simulink model "pwm_thesis"  (R2018a)
settings: Solver=VariableStepAuto  StartTime=0.0  StopTime=5  MaxStep=0.01  RelTol=1e-3
libraries: powerlib x75, simulink x17, powerlib_meascontrol x1
settings Model: Creator=buzaevfedor  LastModifiedBy=buzaevfedor
settings SolverCC: ZeroCrossAlgorithm=Adaptive
settings DebuggingCC: MaxConsecutiveZCsMsg=none  MaskedZcDiagnostic=none

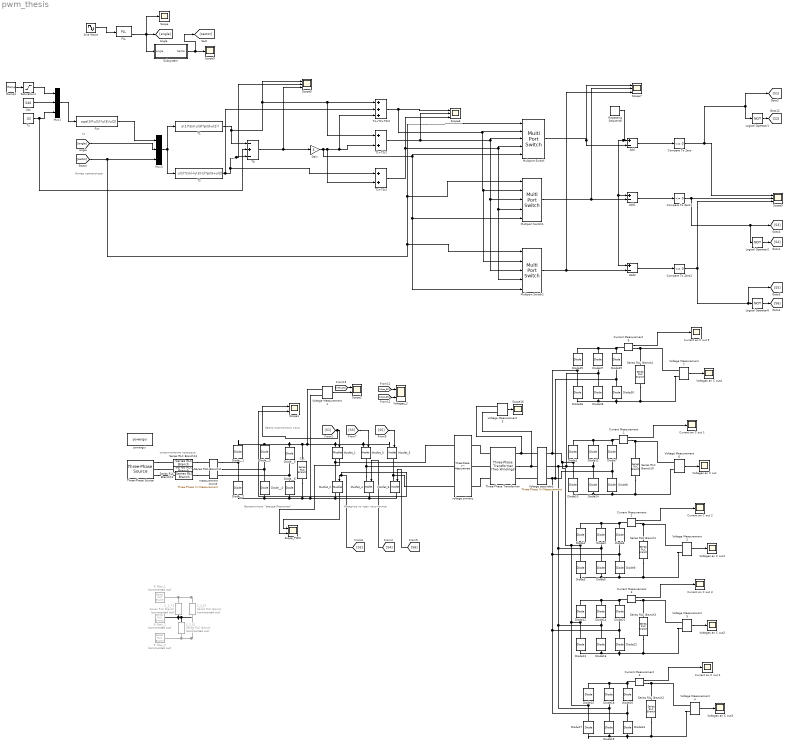
== system pwm_thesis ==
  note: Номер транзистора
  note: wt
  note: Выпрямитель "звезда-Ларионов"
  note: Звено постоянного тока
  note: Инвертор из трех полумостов
  note: сопротивление проводов
  Add : Sum  Inputs=+-
  Add1 : Sum  Inputs=+-
  Add2 : Sum  Inputs=+-
  C_1 : powerlib/Elements/Series RLC Branch  LConnTagsString=__new0  RConnTagsString=__new0  BranchType=C  Resistance=1  Inductance=1e-3  SetiL0=off  InitialCurrent=0  Capacitance=1000e-6  Setx0=off  InitialVoltage=0  Measurements=Branch voltage and current
  C_1_f 2 : powerlib/Elements/Series RLC Branch  Commented=on  LConnTagsString=__new0  RConnTagsString=__new0  BranchType=C  Resistance=1  Inductance=1e-3  SetiL0=off  InitialCurrent=0  Capacitance=1100e-8  Setx0=off  InitialVoltage=0  Measurements=None
  C_2_f2 : powerlib/Elements/Series RLC Branch  Commented=on  LConnTagsString=__new0  RConnTagsString=__new0  BranchType=C  Resistance=1  Inductance=1e-3  SetiL0=off  InitialCurrent=0  Capacitance=1100e-8  Setx0=off  InitialVoltage=0  Measurements=None
  C_3_f2 : powerlib/Elements/Series RLC Branch  Commented=on  LConnTagsString=__new0  RConnTagsString=__new0  BranchType=C  Resistance=1  Inductance=1e-3  SetiL0=off  InitialCurrent=0  Capacitance=1100e-8  Setx0=off  InitialVoltage=0  Measurements=None
  Compare To Zero : simulink/Logic and Bit Operations/Compare To Zero  relop=<=  OutDataTypeStr=boolean
  Compare To Zero1 : simulink/Logic and Bit Operations/Compare To Zero  relop=<=  OutDataTypeStr=boolean
  Compare To Zero2 : simulink/Logic and Bit Operations/Compare To Zero  relop=<=  OutDataTypeStr=boolean
  Current Measurement{1..5} (5 alike) : powerlib/Measurements/Current Measurement  PhasorSimulation=off  OutputType=Complex  PSBequivalent=0
  Current an C out {1..5} (5 alike) : Scope
  Diode{1..30} (30 alike) : powerlib/Power Electronics/Diode  Ron=0.001  Lon=0  Vf=0.8  IC=0  UseSnubber=0  Rs=500  Cs=250e-9  Measurements=off
  Diode__{1..6} (6 alike) : powerlib/Power Electronics/Diode  Ron=0.001  Lon=0  Vf=0.8  IC=0  UseSnubber=0  Rs=500  Cs=250e-9  Measurements=off
  Fcn : Fcn  Expr=sqrt(3)*u(1)*u(3)/u(2)
  Gain : Gain  Gain=.5
  Logical Operator1 : Logic  Operator=NOT  AllPortsSameDT=off  OutDataTypeStr=boolean
  Logical Operator2 : Logic  Operator=NOT  AllPortsSameDT=off  OutDataTypeStr=boolean
  Logical Operator6 : Logic  Operator=NOT  AllPortsSameDT=off  OutDataTypeStr=boolean
  Mosfet_1 : powerlib/Power Electronics/Mosfet  Ron=0.1  Lon=0  Rd=0.01  Vfd=0  IC=0  Rs=1e5  Cs=inf  Measurements=on
  Mosfet_2 : powerlib/Power Electronics/Mosfet  Ron=0.1  Lon=0  Rd=0.01  Vfd=0  IC=0  Rs=1e5  Cs=inf  Measurements=on
  Mosfet_{3..6} (4 alike) : powerlib/Power Electronics/Mosfet  Ron=0.1  Lon=0  Rd=0.01  Vfd=0  IC=0  Rs=1e5  Cs=inf  Measurements=off
  Multiport Switch : MultiPortSwitch  DataPortOrder=Specify indices  Inputs=4  DataPortIndices={[1,6],2,5,[3,4]}  DiagnosticForDefault=Warning
  Multiport Switch1 : MultiPortSwitch  DataPortOrder=Specify indices  Inputs=4  DataPortIndices={[2,3],4,1,[5,6]}  DiagnosticForDefault=Warning
  Multiport Switch2 : MultiPortSwitch  DataPortOrder=Specify indices  Inputs=4  DataPortIndices={[4,5],6,3,[1,2]}  DiagnosticForDefault=Warning
  Mux1 : Mux  Inputs=3
  Mux3 : Mux  Inputs=3
  PLL : powerlib_meascontrol/PLL/PLL  Fmin=45  Par_Init=[0, 50]  ParK=[180, 3200, 1]  TcD=1e-4  MaxRateChangeFreq=12  FilterCutOffFreq=25  Ts=0  AGC=on
      settings: SourceProductName=Simscape Power Systems  SourceProductBaseCode=PS
  R filter_1 : powerlib/Elements/Series RLC Branch  Commented=on  LConnTagsString=__new0  RConnTagsString=__new0  BranchType=R  Resistance=80  Inductance=1e-3  SetiL0=off  InitialCurrent=0  Capacitance=1e-6  Setx0=off  InitialVoltage=0  Measurements=None
  R filter_2 : powerlib/Elements/Series RLC Branch  Commented=on  LConnTagsString=__new0  RConnTagsString=__new0  BranchType=R  Resistance=80  Inductance=1e-3  SetiL0=off  InitialCurrent=0  Capacitance=1e-6  Setx0=off  InitialVoltage=0  Measurements=None
  R filter_3 : powerlib/Elements/Series RLC Branch  Commented=on  LConnTagsString=__new0  RConnTagsString=__new0  BranchType=R  Resistance=80  Inductance=1e-3  SetiL0=off  InitialCurrent=0  Capacitance=1e-6  Setx0=off  InitialVoltage=0  Measurements=None
  Ramp1 : simulink/Sources/Ramp  slope=55  start=0  InitialOutput=0
  Repeating Sequence : simulink/Sources/Repeating Sequence  rep_seq_t=[0 .001]  rep_seq_y=[0 .02]
  Saturation1 : Saturate  UpperLimit=220
  Scope : Scope
  Scope1 : Scope  NumInputPorts=2
  Scope16 : Scope
  Scope2 : Scope  NumInputPorts=2
  Scope3 : Scope
  Scope{5..7,9} (4 alike) : Scope  NumInputPorts=3
  Scope_PWM : Scope  NumInputPorts=2
  Series RLC Branch{1..4,10} (5 alike) : powerlib/Elements/Series RLC Branch  LConnTagsString=__new0  RConnTagsString=__new0  BranchType=C  Resistance=1  Inductance=1e-3  SetiL0=off  InitialCurrent=0  Capacitance=12e-3  Setx0=off  InitialVoltage=0  Measurements=Branch voltage and current
  Series RLC Branch11 : powerlib/Elements/Series RLC Branch  LConnTagsString=__new0  RConnTagsString=__new0  BranchType=RL  Resistance=1  Inductance=1e-3  SetiL0=off  InitialCurrent=0  Capacitance=1e-6  Setx0=off  InitialVoltage=0  Measurements=None
  Series RLC Branch12 : powerlib/Elements/Series RLC Branch  LConnTagsString=__new0  RConnTagsString=__new0  BranchType=RL  Resistance=1  Inductance=1e-3  SetiL0=off  InitialCurrent=0  Capacitance=1e-6  Setx0=off  InitialVoltage=0  Measurements=None
  Series RLC Branch13 : powerlib/Elements/Series RLC Branch  LConnTagsString=__new0  RConnTagsString=__new0  BranchType=RL  Resistance=1  Inductance=1e-3  SetiL0=off  InitialCurrent=0  Capacitance=1e-6  Setx0=off  InitialVoltage=0  Measurements=None
  Sine Wave : Sin  Frequency=2*pi*50  SampleTime=0
  Subsystem : Subsystem
  T0 : Sum  Inputs=-+-
  T1 : Fcn  Expr=u(1)*sin(u(3)*pi/3-u(2))
  T1+T0/2 : Sum  Inputs=2
  T1+T2+T0/2 : Sum  Inputs=+++
  T2 : Fcn  Expr=u(1)*sin(-(u(3)-1)*pi/3+u(2))
  T2+T0/2 : Sum  Inputs=2
  Three-Phase Transformer : powerlib/Elements/Three-Phase Transformer (Two Windings)  Winding1Connection=Yg  Winding2Connection=Yg  CoreType=Three single-phase transformers  SetSaturation=off  Hysteresis=off  DataFile='hysteresis'  SetInitialFlux=off  Measurements=None  UNITS=SI  NominalPower=[8549523 , 50 ]  Winding1=[7.35e+05 0.069 1.108e-03]  Winding2=[14.15e+05 8.86e-4 0.09e-03]  Rm=5980.4  Lm=19.93  L0=0.5  Saturation=[0 0;0.66653 1910.3;277.72 2419.7]  InitialFluxes=[1273.5 -1273.5 1114.3]  MoreParameters=off  BreakLoop=off  DataType=on  TransfoNumber=1
  Three-Phase Source : powerlib/Electrical Sources/Three-Phase Source  InternalConnection=Yg  VoltagePhases=on  Voltage=380  PhaseAngle=0  Voltage_phases=[380 380 380]/sqrt(3)  PhaseAngles_phases=[0 -120 +120]  Frequency=50  NonIdealSource=off  SpecifyImpedance=off  Resistance=0.8929  Inductance=16.58e-3  ShortCircuitLevel=100e6  BaseVoltage=25e3  XRratio=7  BusType=swing  Pref=10e3  Qref=0  Prefabc=[10e3, 10e3, 10e3]  Qrefabc=[0, 0, 0]  Qmin=-inf  Qmax=inf
  Tz : Constant  Value=.02
  Udc : Constant  Value=540
  Voltage Measurement{1..7} (7 alike) : powerlib/Measurements/Voltage Measurement  PhasorSimulation=off  OutputType=Complex  PSBequivalent=0
  Voltage secondary : powerlib/Measurements/Three-Phase V-I Measurement  VoltageMeasurement=phase-to-phase  SetLabelV=on  LabelV=Vabc_B3  Vpu=off  VpuLL=off  CurrentMeasurement=yes  SetLabelI=on  LabelI=Iabc_B3  Ipu=off  Pbase=225e3  Vbase=2400  OutputType=Complex  PhasorSimulation=off  PSBequivalent=0
  Voltages an C out{,1..4} (5 alike) : Scope
  Voltages_2 : Scope  NumInputPorts=2
  measurement source : powerlib/Measurements/Three-Phase V-I Measurement  VoltageMeasurement=phase-to-phase  SetLabelV=on  LabelV=Vabc_B1  Vpu=off  VpuLL=off  CurrentMeasurement=yes  SetLabelI=on  LabelI=Iabc_B1  Ipu=off  Pbase=225e3  Vbase=2400  OutputType=Complex  PhasorSimulation=off  PSBequivalent=0
  powergui : powerlib/powergui  Priority=1  SimulationMode=Continuous  SampleTime=50e-6  frequency=60  Iterations=50  frequencyindice=50  Pbase=100e6  ErrMax=1e-4  UnitsV=kV  UnitsW=MW  buscounter=0  FunctionMessages=off  echomessages=off  EnableUseOfTLC=off  CurrentSourceSwitches=off  DisableSnubberDevices=off  DisableRonSwitches=off  DisableVfSwitches=off  DisplayEquations=off  SolverType=Tustin/Backward Euler (TBE)  Interpol=off  ExternalGateDelay=off  methode=off  Ts=100  x0status=blocks  SPID=on  SwTol=0  HookPort=off  RestoreLinks=warning  ResistiveCurrentMeasurement=off  Frange=[0:2:500]  Ylog=off  Xlog=on  ShowGrid=off  save=off  variable=ZData  structure=0  ZoomFFT=off  StartTime=0.0  cycles=1  DisplayStyle=1  fundamental=60  FreqAxis=off  MaxFrequency=1000  frequencyindicesteady=1  RmsSteady=1  display=off
  "voltage primary " : powerlib/Measurements/Three-Phase V-I Measurement  VoltageMeasurement=phase-to-phase  SetLabelV=on  LabelV=Vabc_B2  Vpu=off  VpuLL=off  CurrentMeasurement=yes  SetLabelI=on  LabelI=Iabc_B2  Ipu=off  Pbase=225e3  Vbase=2400  OutputType=Complex  PhasorSimulation=off  PSBequivalent=0
  wires:
  Voltage Measurement3/1 -> Scope16/1
  Voltage Measurement6/1 -> Voltages an C out/1
  [Vabc_B3] -> Voltages_2/2
  [Vabc_B2] -> Voltages_2/1
  [S6] -> Mosfet_6/1
  [S2] -> Scope1/2, Mosfet_2/1
  [S3] -> Mosfet_3/1
  [S5] -> Mosfet_5/1
  [S1] -> Scope1/1, Mosfet_1/1
  Voltage Measurement1/1 -> Scope2/2
  [Vabc_B1] -> Scope2/1
  Mosfet_1/1 -> Scope_PWM/2
  Mosfet_2/1 -> Scope_PWM/1
  Current Measurement1/1 -> Current an C out 1/1
  Tz/1 -> T0/2, Mux1/3
  Compare To Zero1/1 -> Logical Operator2/1, [S3], Scope9/2
  Add/1 -> Compare To Zero/1
  Udc/1 -> Mux1/2
  Sine Wave/1 -> PLL/1
  Repeating Sequence/1 -> Add2/1, Add1/1, Add/1
  Multiport Switch2/1 -> Add2/2, Scope7/3
  Mux3/1 -> T2/1, T1/1
  T1+T0/2/1 -> Multiport Switch2/3, Multiport Switch1/3, Multiport Switch/3, Scope6/2
  Compare To Zero2/1 -> Scope9/3, [S5], Logical Operator6/1
  Gain/1 -> Multiport Switch2/5, Multiport Switch1/5, Multiport Switch/5, T2+T0/2/2, T1+T0/2/2, T1+T2+T0/2/3
  Multiport Switch/1 -> Add/2, Scope7/1
  Logical Operator1/1 -> [S2]
  T1/1 -> T1+T2+T0/2/1, T1+T0/2/1, Scope5/1, T0/1
  Fcn/1 -> Mux3/1
  Logical Operator6/1 -> [S6]
  Multiport Switch1/1 -> Add1/2, Scope7/2
  PLL/2 -> Scope/1, Subsystem/1(angle), [angle]
  [sector] -> Multiport Switch2/1, Multiport Switch1/1, Multiport Switch/1, Mux3/3
  T2/1 -> T1+T2+T0/2/2, T2+T0/2/1, Scope5/2, T0/3
  Subsystem/1(Sector) -> [sector], Scope3/1
  Add1/1 -> Compare To Zero1/1
  Logical Operator2/1 -> [S4]
  Mux1/1 -> Fcn/1
  Compare To Zero/1 -> Logical Operator1/1, [S1], Scope9/1
  [angle] -> Mux3/2
  T2+T0/2/1 -> Multiport Switch2/4, Multiport Switch1/4, Multiport Switch/4, Scope6/3
  T1+T2+T0/2/1 -> Multiport Switch2/2, Multiport Switch1/2, Multiport Switch/2, Scope6/1
  Add2/1 -> Compare To Zero2/1
  T0/1 -> Scope5/3, Gain/1
  [S4] -> Mosfet_4/1
  Ramp1/1 -> Saturation1/1
  Saturation1/1 -> Mux1/1
  Current Measurement2/1 -> Current an C out 2/1
  Voltage Measurement2/1 -> Voltages an C out1/1
  Voltage Measurement4/1 -> Voltages an C out3/1
  Current Measurement4/1 -> Current an C out 4/1
  Current Measurement3/1 -> Current an C out 3/1
  Voltage Measurement5/1 -> Voltages an C out2/1
  Current Measurement5/1 -> Current an C out 5/1
  Voltage Measurement7/1 -> Voltages an C out4/1
  connections:
  Diode8/LConn1 -- Diode10/LConn1 -- Diode24/LConn1 -- Voltage Measurement6/LConn2 -- Series RLC Branch10/RConn1
  Diode15/LConn1 -- Diode25/LConn1 -- Diode26/RConn1 -- Voltage secondary/RConn1 -- Diode10/RConn1 -- Diode1/LConn1 -- Diode2/LConn1 -- Diode3/RConn1 -- Diode12/LConn1 -- Diode13/RConn1 -- Diode17/RConn1
  Diode__6/RConn1 -- measurement source/RConn3 -- Diode__5/LConn1
  Mosfet_6/RConn1 -- Diode__2/LConn1 -- Diode__4/LConn1 -- Diode__6/LConn1 -- C_1/RConn1 -- Voltage Measurement1/LConn2 -- Mosfet_2/RConn1 -- Mosfet_4/RConn1
  Diode1/RConn1 -- Current Measurement1/LConn1 -- Diode7/RConn1 -- Diode11/RConn1
  Diode18/LConn1 -- Voltage secondary/RConn2 -- Diode27/LConn1 -- Diode28/RConn1 -- Diode24/RConn1 -- Diode11/LConn1 -- Diode4/LConn1 -- Diode5/RConn1 -- Diode14/LConn1 -- Diode16/RConn1 -- Diode19/RConn1
  Diode__5/RConn1 -- C_1/LConn1 -- Mosfet_1/LConn1 -- Mosfet_3/LConn1 -- Mosfet_5/LConn1 -- Voltage Measurement1/LConn1 -- Diode__1/RConn1 -- Diode__3/RConn1
  Voltage Measurement3/LConn2 -- Three-Phase Transformer/RConn2 -- Voltage secondary/LConn2
  Diode__4/RConn1 -- measurement source/RConn2 -- Diode__3/LConn1
  Voltage Measurement3/LConn1 -- Three-Phase Transformer/RConn1 -- Voltage secondary/LConn1
  Diode__1/LConn1 -- measurement source/RConn1 -- Diode__2/RConn1
  Diode20/LConn1 -- Voltage secondary/RConn3 -- Diode29/LConn1 -- Diode30/RConn1 -- Diode8/RConn1 -- Diode7/LConn1 -- Diode6/LConn1 -- Diode9/RConn1 -- Diode21/LConn1 -- Diode22/RConn1 -- Diode23/RConn1
  Three-Phase Transformer/RConn3 -- Voltage secondary/LConn3
  Three-Phase Transformer/LConn3 -- "voltage primary "/RConn3
  Series RLC Branch11/RConn1 -- measurement source/LConn2
  Series RLC Branch13/RConn1 -- measurement source/LConn1
  Three-Phase Transformer/LConn2 -- "voltage primary "/RConn2
  Three-Phase Transformer/LConn1 -- "voltage primary "/RConn1
  Series RLC Branch12/RConn1 -- measurement source/LConn3
  Three-Phase Source/RConn2 -- Series RLC Branch11/LConn1
  Three-Phase Source/RConn1 -- Series RLC Branch13/LConn1
  Three-Phase Source/RConn3 -- Series RLC Branch12/LConn1
  Current Measurement1/RConn1 -- Voltage Measurement6/LConn1 -- Series RLC Branch10/LConn1
  Mosfet_2/LConn1 -- "voltage primary "/LConn1 -- Mosfet_1/RConn1
  Mosfet_6/LConn1 -- "voltage primary "/LConn3 -- Mosfet_5/RConn1
  Mosfet_4/LConn1 -- "voltage primary "/LConn2 -- Mosfet_3/RConn1
  C_3_f2/LConn1 -- C_1_f 2/LConn1 -- R filter_1/LConn1
  C_3_f2/RConn1 -- R filter_3/LConn1 -- C_2_f2/RConn1
  C_1_f 2/RConn1 -- R filter_2/LConn1 -- C_2_f2/LConn1
  Diode9/LConn1 -- Series RLC Branch1/RConn1 -- Voltage Measurement2/LConn2 -- Diode5/LConn1 -- Diode3/LConn1
  Diode2/RConn1 -- Diode4/RConn1 -- Diode6/RConn1 -- Current Measurement2/LConn1
  Current Measurement2/RConn1 -- Series RLC Branch1/LConn1 -- Voltage Measurement2/LConn1
  Diode22/LConn1 -- Series RLC Branch3/RConn1 -- Voltage Measurement5/LConn2 -- Diode16/LConn1 -- Diode13/LConn1
  Diode12/RConn1 -- Diode14/RConn1 -- Diode21/RConn1 -- Current Measurement3/LConn1
  Current Measurement3/RConn1 -- Series RLC Branch3/LConn1 -- Voltage Measurement5/LConn1
  Diode19/LConn1 -- Diode23/LConn1 -- Voltage Measurement4/LConn2 -- Series RLC Branch2/RConn1 -- Diode17/LConn1
  Diode20/RConn1 -- Diode15/RConn1 -- Diode18/RConn1 -- Current Measurement4/LConn1
  Series RLC Branch2/LConn1 -- Current Measurement4/RConn1 -- Voltage Measurement4/LConn1
  Diode30/LConn1 -- Series RLC Branch4/RConn1 -- Voltage Measurement7/LConn2 -- Diode28/LConn1 -- Diode26/LConn1
  Diode25/RConn1 -- Diode27/RConn1 -- Diode29/RConn1 -- Current Measurement5/LConn1
  Current Measurement5/RConn1 -- Series RLC Branch4/LConn1 -- Voltage Measurement7/LConn1

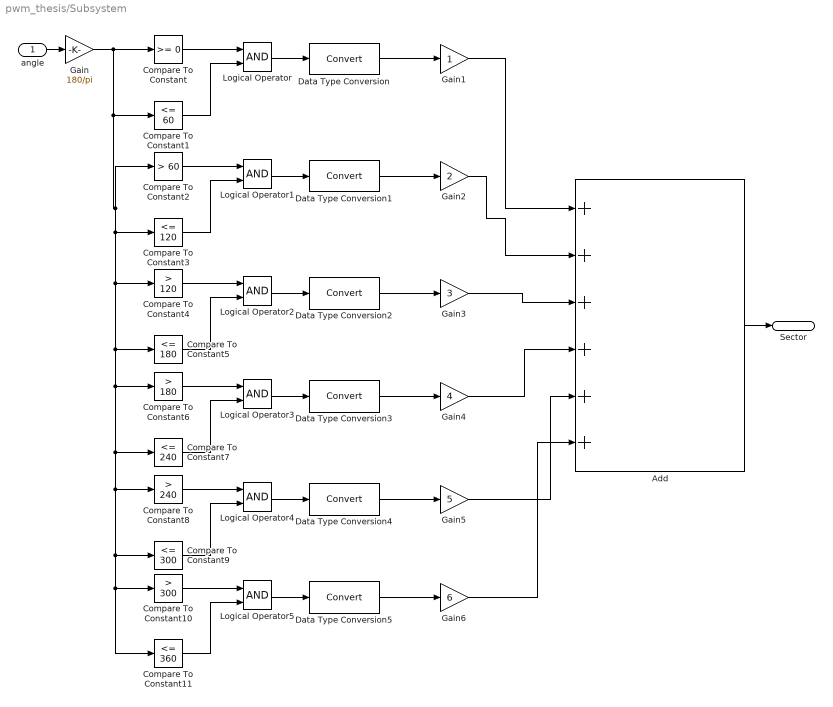
== system pwm_thesis/Subsystem ==
  angle : Inport
  Add : Sum  Inputs=6
  Compare To Constant : simulink/Logic and Bit Operations/Compare To Constant  relop=>=  const=0  OutDataTypeStr=boolean
  Compare To Constant1 : simulink/Logic and Bit Operations/Compare To Constant  relop=<=  const=60  OutDataTypeStr=boolean
  Compare To Constant10 : simulink/Logic and Bit Operations/Compare To Constant  relop=>  const=300  OutDataTypeStr=boolean
  Compare To Constant11 : simulink/Logic and Bit Operations/Compare To Constant  relop=<=  const=360  OutDataTypeStr=boolean
  Compare To Constant2 : simulink/Logic and Bit Operations/Compare To Constant  relop=>  const=60  OutDataTypeStr=boolean
  Compare To Constant3 : simulink/Logic and Bit Operations/Compare To Constant  relop=<=  const=120  OutDataTypeStr=boolean
  Compare To Constant4 : simulink/Logic and Bit Operations/Compare To Constant  relop=>  const=120  OutDataTypeStr=boolean
  Compare To Constant5 : simulink/Logic and Bit Operations/Compare To Constant  relop=<=  const=180  OutDataTypeStr=boolean
  Compare To Constant6 : simulink/Logic and Bit Operations/Compare To Constant  relop=>  const=180  OutDataTypeStr=boolean
  Compare To Constant7 : simulink/Logic and Bit Operations/Compare To Constant  relop=<=  const=240  OutDataTypeStr=boolean
  Compare To Constant8 : simulink/Logic and Bit Operations/Compare To Constant  relop=>  const=240  OutDataTypeStr=boolean
  Compare To Constant9 : simulink/Logic and Bit Operations/Compare To Constant  relop=<=  const=300  OutDataTypeStr=boolean
  Data Type Conversion{,1..5} (6 alike) : DataTypeConversion
  Gain : Gain  Gain=180/pi
  Gain1 : Gain
  Gain2 : Gain  Gain=2
  Gain3 : Gain  Gain=3
  Gain4 : Gain  Gain=4
  Gain5 : Gain  Gain=5
  Gain6 : Gain  Gain=6
  Logical Operator{,1..5} (6 alike) : Logic  AllPortsSameDT=off  OutDataTypeStr=boolean
  Sector : Outport
  wires:
  angle/1 -> Gain/1
  Compare To Constant/1 -> Logical Operator/1
  Compare To Constant1/1 -> Logical Operator/2
  Logical Operator/1 -> Data Type Conversion/1
  Data Type Conversion/1 -> Gain1/1
  Data Type Conversion1/1 -> Gain2/1
  Logical Operator1/1 -> Data Type Conversion1/1
  Compare To Constant3/1 -> Logical Operator1/2
  Compare To Constant2/1 -> Logical Operator1/1
  Compare To Constant4/1 -> Logical Operator2/1
  Compare To Constant5/1 -> Logical Operator2/2
  Logical Operator2/1 -> Data Type Conversion2/1
  Data Type Conversion2/1 -> Gain3/1
  Data Type Conversion3/1 -> Gain4/1
  Logical Operator3/1 -> Data Type Conversion3/1
  Compare To Constant7/1 -> Logical Operator3/2
  Compare To Constant6/1 -> Logical Operator3/1
  Compare To Constant8/1 -> Logical Operator4/1
  Compare To Constant9/1 -> Logical Operator4/2
  Logical Operator4/1 -> Data Type Conversion4/1
  Data Type Conversion4/1 -> Gain5/1
  Data Type Conversion5/1 -> Gain6/1
  Logical Operator5/1 -> Data Type Conversion5/1
  Compare To Constant11/1 -> Logical Operator5/2
  Compare To Constant10/1 -> Logical Operator5/1
  Gain/1 -> Compare To Constant5/1, Compare To Constant6/1, Compare To Constant7/1, Compare To Constant10/1, Compare To Constant11/1, Compare To Constant9/1, Compare To Constant8/1, Compare To Constant4/1, Compare To Constant3/1, Compare To Constant2/1, Compare To Constant1/1, Compare To Constant/1
  Gain1/1 -> Add/1
  Gain2/1 -> Add/2
  Gain3/1 -> Add/3
  Gain4/1 -> Add/4
  Gain5/1 -> Add/5
  Gain6/1 -> Add/6
  Add/1 -> Sector/1
